simulink model "gimbal_cold_compensation_135ff_v4"  (R2025a)
settings: Solver=FixedStepDiscrete  StartTime=0.0  StopTime=20  FixedStep=0.01  RelTol=1e-3
undefined symbols (not defined in the file or in its folder): PAN_TARGET_DEG, TILT_TARGET_DEG
settings Model: Creator=polad  LastModifiedBy=polad

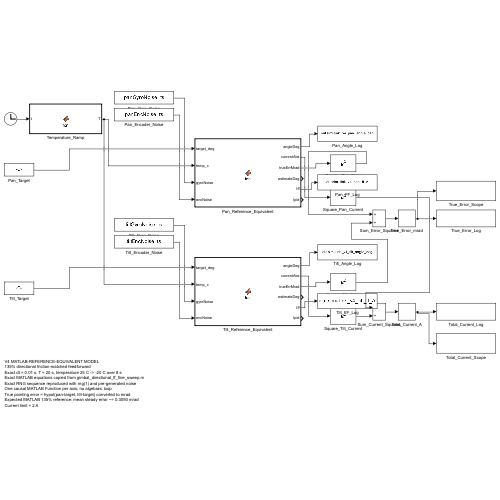
[thumbnail: Simulink's stored preview of the top-level diagram]
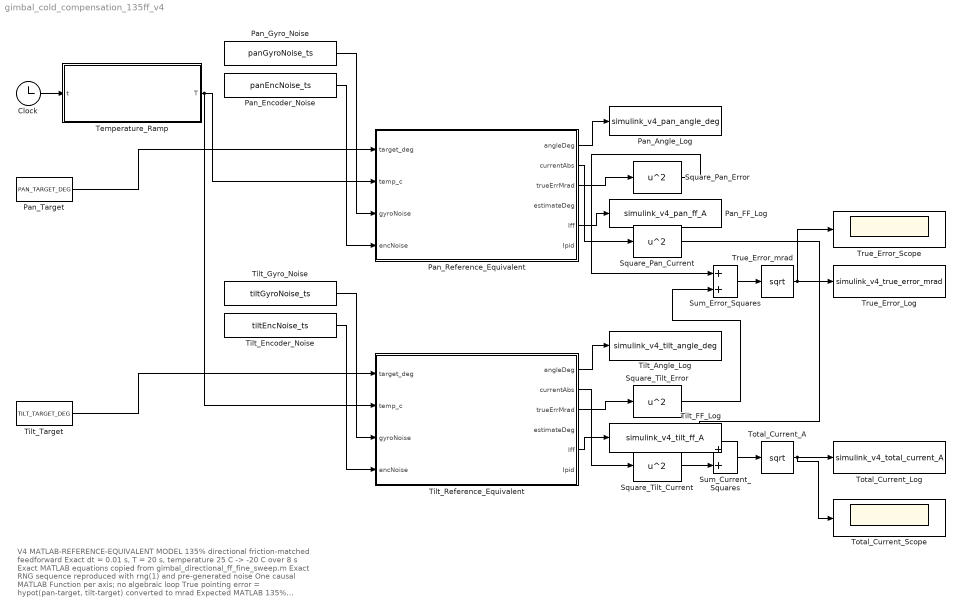
== system gimbal_cold_compensation_135ff_v4 ==
  note: V4 MATLAB-REFERENCE-EQUIVALENT MODEL
      | 135% directional friction-matched feedforward
      | Exact dt = 0.01 s, T = 20 s, temperature 25 C -> -20 C over 8 s
      | Exact MATLAB equations copied from gimbal_directional_ff_fine_sweep.m
      | Exact RNG sequence reproduced with rng(1) and pre-generated noise
      | One causal MATLAB Function per axis; no algebraic loop
      | True pointing error = hypot(pan-target, tilt-target) converted to mrad
      | Expected MATLAB 135% reference: mean steady error ~= 0.3093 mrad
      | Current limit = 2 A
  Clock : Clock
  Pan_Angle_Log : ToWorkspace  VariableName=simulink_v4_pan_angle_deg  SaveFormat=Timeseries  SampleTime=-1
  Pan_Encoder_Noise : FromWorkspace  VariableName=panEncNoise_ts
  Pan_FF_Log : ToWorkspace  VariableName=simulink_v4_pan_ff_A  SaveFormat=Timeseries  SampleTime=-1
  Pan_Gyro_Noise : FromWorkspace  VariableName=panGyroNoise_ts
  Pan_Reference_Equivalent : MATLAB Function  TreatAsAtomicUnit=on
  Pan_Target : Constant  Value=PAN_TARGET_DEG
  Square_Pan_Current : Math  Operator=square
  Square_Pan_Error : Math  Operator=square
  Square_Tilt_Current : Math  Operator=square
  Square_Tilt_Error : Math  Operator=square
  Sum_Current_Squares : Sum
  Sum_Error_Squares : Sum
  Temperature_Ramp : MATLAB Function  TreatAsAtomicUnit=on
  Tilt_Angle_Log : ToWorkspace  VariableName=simulink_v4_tilt_angle_deg  SaveFormat=Timeseries  SampleTime=-1
  Tilt_Encoder_Noise : FromWorkspace  VariableName=tiltEncNoise_ts
  Tilt_FF_Log : ToWorkspace  VariableName=simulink_v4_tilt_ff_A  SaveFormat=Timeseries  SampleTime=-1
  Tilt_Gyro_Noise : FromWorkspace  VariableName=tiltGyroNoise_ts
  Tilt_Reference_Equivalent : MATLAB Function  TreatAsAtomicUnit=on
  Tilt_Target : Constant  Value=TILT_TARGET_DEG
  Total_Current_A : Sqrt
  Total_Current_Log : ToWorkspace  VariableName=simulink_v4_total_current_A  SaveFormat=Timeseries  SampleTime=-1
  Total_Current_Scope : Scope
  True_Error_Log : ToWorkspace  VariableName=simulink_v4_true_error_mrad  SaveFormat=Timeseries  SampleTime=-1
  True_Error_Scope : Scope
  True_Error_mrad : Sqrt
  wires:
  Clock/1 -> Temperature_Ramp/1(t)
  Temperature_Ramp/1(T) -> Pan_Reference_Equivalent/2(temp_c), Tilt_Reference_Equivalent/2(temp_c)
  Pan_Target/1 -> Pan_Reference_Equivalent/1(target_deg)
  Tilt_Target/1 -> Tilt_Reference_Equivalent/1(target_deg)
  Pan_Gyro_Noise/1 -> Pan_Reference_Equivalent/3(gyroNoise)
  Pan_Encoder_Noise/1 -> Pan_Reference_Equivalent/4(encNoise)
  Tilt_Gyro_Noise/1 -> Tilt_Reference_Equivalent/3(gyroNoise)
  Tilt_Encoder_Noise/1 -> Tilt_Reference_Equivalent/4(encNoise)
  Pan_Reference_Equivalent/3(trueErrMrad) -> Square_Pan_Error/1
  Tilt_Reference_Equivalent/3(trueErrMrad) -> Square_Tilt_Error/1
  Square_Pan_Error/1 -> Sum_Error_Squares/1
  Square_Tilt_Error/1 -> Sum_Error_Squares/2
  Sum_Error_Squares/1 -> True_Error_mrad/1
  True_Error_mrad/1 -> True_Error_Log/1, True_Error_Scope/1
  Pan_Reference_Equivalent/2(currentAbs) -> Square_Pan_Current/1
  Tilt_Reference_Equivalent/2(currentAbs) -> Square_Tilt_Current/1
  Square_Pan_Current/1 -> Sum_Current_Squares/1
  Square_Tilt_Current/1 -> Sum_Current_Squares/2
  Sum_Current_Squares/1 -> Total_Current_A/1
  Total_Current_A/1 -> Total_Current_Log/1, Total_Current_Scope/1
  Pan_Reference_Equivalent/1(angleDeg) -> Pan_Angle_Log/1
  Tilt_Reference_Equivalent/1(angleDeg) -> Tilt_Angle_Log/1
  Pan_Reference_Equivalent/5(Iff) -> Pan_FF_Log/1
  Tilt_Reference_Equivalent/5(Iff) -> Tilt_FF_Log/1

== matlab function gimbal_cold_compensation_135ff_v4/Pan_Reference_Equivalent ==
  data: target_deg input; angleDeg output; temp_c input; gyroNoise input; encNoise input; currentAbs output; trueErrMrad output; estimateDeg output; Iff output; Ipid output
function [angleDeg,currentAbs,trueErrMrad,estimateDeg,Iff,Ipid]=fcn(target_deg,temp_c,gyroNoise,encNoise)
                                                                                                        % Exact reference-equivalent discrete axis update.                                                       
                                                                                                        % State persists between 0.01 s simulation steps.                                                        
                                                                                                        persistent kf_angle kf_bias P pid_integral pid_prev true_angle true_vel                                  
                                                                                                        if isempty(kf_angle)                                                                                     
                                                                                                            kf_angle=0;                                                                                          
                                                                                                            kf_bias=0;                                                                                           
                                                                                                            P=[1 0;0 1];                                                                                         
                                                                                                            pid_integral=0;                                                                                      
                                                                                                            pid_prev=0;                                                                                          
                                                                                                            true_angle=0;                                                                                        
                                                                                                            true_vel=0;                                                                                          
                                                                                                        end                                                                                                      
                                                                                                                                                                                                                 
                                                                                                        % Exact constants from gimbal_directional_ff_fine_sweep.m                                                
                                                                                                        dt=0.01;                                                                                                 
                                                                                                        KP=2.5; KI=0.8; KD=0.05;                                                                                 
                                                                                                        PID_OUT_MAX=1.5; PID_INT_MAX=0.5;                                                                        
                                                                                                        QA_BASE=0.001; QB_BASE=0.003; R_MEAS=0.03;                                                               
                                                                                                        J=0.006; DAMP=0.35; FRIC_SCALE=9.0;                                                                      
                                                                                                                                                                                                                 
                                                                                                        % Simulated sensors -- noise is supplied externally in the exact MATLAB order.                           
                                                                                                        gyro_bias_true=0.15*(25-temp_c)*0.03;                                                                    
                                                                                                        gyro_reading=true_vel+gyro_bias_true+gyroNoise;                                                          
                                                                                                        enc_reading=true_angle+encNoise;                                                                         
                                                                                                                                                                                                                 
                                                                                                        % Kalman predict                                                                                         
                                                                                                        rate=gyro_reading-kf_bias;                                                                               
                                                                                                        kf_angle=kf_angle+dt*rate;                                                                               
                                                                                                        dT=abs(temp_c-25);                                                                                       
                                                                                                        scale=1+0.01*dT;                                                                                         
                                                                                                        qA=QA_BASE*scale;                                                                                        
                                                                                                        qB=QB_BASE*scale;                                                                                        
                                                                                                        P00=P(1,1)+dt*(dt*P(2,2)-P(1,2)-P(2,1)+qA);                                                              
                                                                                                        P01=P(1,2)-dt*P(2,2);                                                                                    
                                                                                                        P10=P(2,1)-dt*P(2,2);                                                                                    
                                                                                                        P11=P(2,2)+qB*dt;                                                                                        
                                                                                                        P=[P00 P01;P10 P11];                                                                                     
                                                                                                                                                                                                                 
                                                                                                        % Kalman update                                                                                          
                                                                                                        y=enc_reading-kf_angle;                                                                                  
                                                                                                        S=P(1,1)+R_MEAS;                                                                                         
                                                                                                        K0=P(1,1)/S;                                                                                             
                                                                                                        K1=P(2,1)/S;                                                                                             
                                                                                                        kf_angle=kf_angle+K0*y;                                                                                  
                                                                                                        kf_bias=kf_bias+K1*y;                                                                                    
                                                                                                        p00t=P(1,1);                                                                                             
                                                                                                        p01t=P(1,2);                                                                                             
                                                                                                        P(1,1)=P(1,1)-K0*p00t;                                                                                   
                                                                                                        P(1,2)=P(1,2)-K0*p01t;                                                                                   
                                                                                                        P(2,1)=P(2,1)-K1*p00t;                                                                                   
                                                                                                        P(2,2)=P(2,2)-K1*p01t;                                                                                   
                                                                                                                                                                                                                 
                                                                                                        % PID                                                                                                    
                                                                                                        err=target_deg-kf_angle;                                                                                 
                                                                                                        pid_integral=pid_integral+err*dt;                                                                        
                                                                                                        pid_integral=max(-PID_INT_MAX,min(PID_INT_MAX,pid_integral));                                            
                                                                                                        deriv=(err-pid_prev)/dt;                                                                                 
                                                                                                        pid_prev=err;                                                                                            
                                                                                                        Ipid=KP*err+KI*pid_integral+KD*deriv;                                                                    
                                                                                                        Ipid=max(-PID_OUT_MAX,min(PID_OUT_MAX,Ipid));                                                            
                                                                                                                                                                                                                 
                                                                                                        % Directional friction-matched feedforward, 135%%                                                        
                                                                                                        FF_A=0.05;                                                                                               
                                                                                                        FF_B=-0.0025;                                                                                            
                                                                                                        FF_C=0.00004;                                                                                            
                                                                                                        base=FF_A+FF_B*temp_c+FF_C*temp_c*temp_c;                                                                
                                                                                                        base=max(0,base);                                                                                        
                                                                                                        frictionCurrent=base*9.0;                                                                                
                                                                                                        if abs(err)<1e-6                                                                                         
                                                                                                            direction=0;                                                                                         
                                                                                                        else                                                                                                     
                                                                                                            direction=sign(err);                                                                                 
                                                                                                        end                                                                                                      
                                                                                                        Iff=1.35*frictionCurrent*0.6*direction;                                                                  
                                                                                                        Icmd=max(-2,min(2,Ipid+Iff));                                                                            
                                                                                                                                                                                                                 
                                                                                                        % Exact plant physics                                                                                    
                                                                                                        thresh=base*FRIC_SCALE;                                                                                  
                                                                                                        if abs(true_vel)<0.05                                                                                    
                                                                                                            if abs(Icmd)<=thresh                                                                                 
                                                                                                                fric=-Icmd;                                                                                      
                                                                                                            else                                                                                                 
                                                                                                                fric=-sign(Icmd)*thresh*0.7;                                                                     
                                                                                                            end                                                                                                  
                                                                                                        else                                                                                                     
                                                                                                            fric=-sign(true_vel)*thresh*0.6;                                                                     
                                                                                                        end                                                                                                      
                                                                                                        net=Icmd+fric-DAMP*true_vel;                                                                             
                                                                                                        true_vel=true_vel+(net/J)*dt;                                                                            
                                                                                                        true_angle=true_angle+true_vel*dt;                                                                       
                                                                                                                                                                                                                 
                                                                                                        % Outputs                                                                                                
                                                                                                        angleDeg=true_angle;                                                                                     
                                                                                                        currentAbs=abs(Icmd);                                                                                    
                                                                                                        trueErrMrad=hypot(true_angle-target_deg,0)*pi/180*1000;                                                  
                                                                                                        estimateDeg=kf_angle;                                                                                    
                                                                                                        end

== matlab function gimbal_cold_compensation_135ff_v4/Temperature_Ramp ==
  data: t input; T output
function T=fcn(t) 
                 if t<=8           
                     T=25-(45/8)*t;
                 else              
                     T=-20;        
                 end               
                 end

== matlab function gimbal_cold_compensation_135ff_v4/Tilt_Reference_Equivalent ==
  data: target_deg input; angleDeg output; temp_c input; gyroNoise input; encNoise input; currentAbs output; trueErrMrad output; estimateDeg output; Iff output; Ipid output
function [angleDeg,currentAbs,trueErrMrad,estimateDeg,Iff,Ipid]=fcn(target_deg,temp_c,gyroNoise,encNoise)
                                                                                                        % Exact reference-equivalent discrete axis update.                                                       
                                                                                                        % State persists between 0.01 s simulation steps.                                                        
                                                                                                        persistent kf_angle kf_bias P pid_integral pid_prev true_angle true_vel                                  
                                                                                                        if isempty(kf_angle)                                                                                     
                                                                                                            kf_angle=0;                                                                                          
                                                                                                            kf_bias=0;                                                                                           
                                                                                                            P=[1 0;0 1];                                                                                         
                                                                                                            pid_integral=0;                                                                                      
                                                                                                            pid_prev=0;                                                                                          
                                                                                                            true_angle=0;                                                                                        
                                                                                                            true_vel=0;                                                                                          
                                                                                                        end                                                                                                      
                                                                                                                                                                                                                 
                                                                                                        % Exact constants from gimbal_directional_ff_fine_sweep.m                                                
                                                                                                        dt=0.01;                                                                                                 
                                                                                                        KP=2.5; KI=0.8; KD=0.05;                                                                                 
                                                                                                        PID_OUT_MAX=1.5; PID_INT_MAX=0.5;                                                                        
                                                                                                        QA_BASE=0.001; QB_BASE=0.003; R_MEAS=0.03;                                                               
                                                                                                        J=0.006; DAMP=0.35; FRIC_SCALE=9.0;                                                                      
                                                                                                                                                                                                                 
                                                                                                        % Simulated sensors -- noise is supplied externally in the exact MATLAB order.                           
                                                                                                        gyro_bias_true=0.15*(25-temp_c)*0.03;                                                                    
                                                                                                        gyro_reading=true_vel+gyro_bias_true+gyroNoise;                                                          
                                                                                                        enc_reading=true_angle+encNoise;                                                                         
                                                                                                                                                                                                                 
                                                                                                        % Kalman predict                                                                                         
                                                                                                        rate=gyro_reading-kf_bias;                                                                               
                                                                                                        kf_angle=kf_angle+dt*rate;                                                                               
                                                                                                        dT=abs(temp_c-25);                                                                                       
                                                                                                        scale=1+0.01*dT;                                                                                         
                                                                                                        qA=QA_BASE*scale;                                                                                        
                                                                                                        qB=QB_BASE*scale;                                                                                        
                                                                                                        P00=P(1,1)+dt*(dt*P(2,2)-P(1,2)-P(2,1)+qA);                                                              
                                                                                                        P01=P(1,2)-dt*P(2,2);                                                                                    
                                                                                                        P10=P(2,1)-dt*P(2,2);                                                                                    
                                                                                                        P11=P(2,2)+qB*dt;                                                                                        
                                                                                                        P=[P00 P01;P10 P11];                                                                                     
                                                                                                                                                                                                                 
                                                                                                        % Kalman update                                                                                          
                                                                                                        y=enc_reading-kf_angle;                                                                                  
                                                                                                        S=P(1,1)+R_MEAS;                                                                                         
                                                                                                        K0=P(1,1)/S;                                                                                             
                                                                                                        K1=P(2,1)/S;                                                                                             
                                                                                                        kf_angle=kf_angle+K0*y;                                                                                  
                                                                                                        kf_bias=kf_bias+K1*y;                                                                                    
                                                                                                        p00t=P(1,1);                                                                                             
                                                                                                        p01t=P(1,2);                                                                                             
                                                                                                        P(1,1)=P(1,1)-K0*p00t;                                                                                   
                                                                                                        P(1,2)=P(1,2)-K0*p01t;                                                                                   
                                                                                                        P(2,1)=P(2,1)-K1*p00t;                                                                                   
                                                                                                        P(2,2)=P(2,2)-K1*p01t;                                                                                   
                                                                                                                                                                                                                 
                                                                                                        % PID                                                                                                    
                                                                                                        err=target_deg-kf_angle;                                                                                 
                                                                                                        pid_integral=pid_integral+err*dt;                                                                        
                                                                                                        pid_integral=max(-PID_INT_MAX,min(PID_INT_MAX,pid_integral));                                            
                                                                                                        deriv=(err-pid_prev)/dt;                                                                                 
                                                                                                        pid_prev=err;                                                                                            
                                                                                                        Ipid=KP*err+KI*pid_integral+KD*deriv;                                                                    
                                                                                                        Ipid=max(-PID_OUT_MAX,min(PID_OUT_MAX,Ipid));                                                            
                                                                                                                                                                                                                 
                                                                                                        % Directional friction-matched feedforward, 135%%                                                        
                                                                                                        FF_A=0.05;                                                                                               
                                                                                                        FF_B=-0.0025;                                                                                            
                                                                                                        FF_C=0.00004;                                                                                            
                                                                                                        base=FF_A+FF_B*temp_c+FF_C*temp_c*temp_c;                                                                
                                                                                                        base=max(0,base);                                                                                        
                                                                                                        frictionCurrent=base*9.0;                                                                                
                                                                                                        if abs(err)<1e-6                                                                                         
                                                                                                            direction=0;                                                                                         
                                                                                                        else                                                                                                     
                                                                                                            direction=sign(err);                                                                                 
                                                                                                        end                                                                                                      
                                                                                                        Iff=1.35*frictionCurrent*0.6*direction;                                                                  
                                                                                                        Icmd=max(-2,min(2,Ipid+Iff));                                                                            
                                                                                                                                                                                                                 
                                                                                                        % Exact plant physics                                                                                    
                                                                                                        thresh=base*FRIC_SCALE;                                                                                  
                                                                                                        if abs(true_vel)<0.05                                                                                    
                                                                                                            if abs(Icmd)<=thresh                                                                                 
                                                                                                                fric=-Icmd;                                                                                      
                                                                                                            else                                                                                                 
                                                                                                                fric=-sign(Icmd)*thresh*0.7;                                                                     
                                                                                                            end                                                                                                  
                                                                                                        else                                                                                                     
                                                                                                            fric=-sign(true_vel)*thresh*0.6;                                                                     
                                                                                                        end                                                                                                      
                                                                                                        net=Icmd+fric-DAMP*true_vel;                                                                             
                                                                                                        true_vel=true_vel+(net/J)*dt;                                                                            
                                                                                                        true_angle=true_angle+true_vel*dt;                                                                       
                                                                                                                                                                                                                 
                                                                                                        % Outputs                                                                                                
                                                                                                        angleDeg=true_angle;                                                                                     
                                                                                                        currentAbs=abs(Icmd);                                                                                    
                                                                                                        trueErrMrad=hypot(true_angle-target_deg,0)*pi/180*1000;                                                  
                                                                                                        estimateDeg=kf_angle;                                                                                    
                                                                                                        end
